simulink model "SquatTrotClimbRefinedDesign_Energy"  (R2025b)
settings: Solver=ode45  StartTime=0.0  StopTime=200  MaxStep=0.1  RelTol=0.01  AbsTol=0.01  EnableMultiTasking=on
undefined symbols (not defined in the file): waypoints, X, Y, Z
libraries: nesl_utility x26, Quadruped_Lib x22, sm_lib x19, slpidlib x2, robotalgslib x1, sharedtransform x1
(part 3 of 3)

== matlab function SquatTrotClimbRefinedDesign_Energy/Rear_left_gait/MATLAB Function2 ==
  data: t input; leg_id input; q_hip output; mode_cmd input
function q_hip = hip_motion_all_legs(t, leg_id, mode_cmd)
    T_squat_start = 101;
    T_walk_start  = 129;
    
    % --- [NEW] Absolute time node for ending the walk ---
    T_walk_end    = 169;  % Start braking and retracting legs exactly at 170 seconds
    
    if (mode_cmd == 1) || (t < T_squat_start)
        q_hip = 0; return;
    end
    
    % Phase 1: Squat and stand (102s - 130s)
    if t < T_walk_start
        tau = t - T_squat_start;
        q_stand = 0; q_squat = deg2rad(35);
        T1=3; T2=15; T3=3;
        
        if tau < T1
            u = tau/T1; 
            q_hip = (1-u)*q_stand + u*q_squat;
        elseif tau < T1+T2
            q_hip = q_squat;
        elseif tau < T1+T2+T3
            u = (tau-(T1+T2))/T3; 
            q_hip = (1-u)*q_squat + u*q_stand;
        else
            q_hip = 0; 
        end
        return;
    end
    
    % Phase 2: Walking logic (130s+)
    % Relative time starting from 130s
    t_phase2 = t - T_walk_start;
    
    % ================= Tunables (Hip) =================
    ang_hip_crouch = deg2rad(30);    
    hip_swing_amp  = deg2rad(9);     
    
    ang_fwd  = ang_hip_crouch - hip_swing_amp;  
    ang_back = ang_hip_crouch + hip_swing_amp;  
    
    % ================= Timing =================
    T_crouch = 2.0;              
    T_hold   = 3.0;              
    T_ramp   = 2.0;              
    T_cycle  = 1.8;
    duty     = 0.50;             
    
    % --- [NEW] Braking and recovery time periods ---
    T_ramp_down = 2.0;    % 170s - 172s: Take 2 seconds to slowly reduce stride amplitude to 0
    T_recover   = 3.0;    % 172s - 175s: After legs stop, take 3 seconds to smoothly stand up straight (return to 0 degrees)
    
    % ================= Phase offsets =================
    phase_offset = [0.0, 0.5, 0.0, 0.5];
    phi = phase_offset(leg_id + 1);
    
    % ================= Smooth interpolators =================
    smooth = @(x) (1 - cos(x * pi)) / 2;
    
    % ==========================================================
    % Stage 1 & 2: Crouch & Hold (relative to 130s) -> (130s ~ 135s)
    % ==========================================================
    if t_phase2 < T_crouch + T_hold
        s = smooth(min(t_phase2 / T_crouch, 1.0));
        q_hip = s * ang_hip_crouch;
        return;
    end
    
    % ==========================================================
    % Stage 3: Trot & Stop (All motions after 135s)
    % ==========================================================
    t_trot = t_phase2 - T_crouch - T_hold;
    phase = mod(t_trot / T_cycle + phi, 1.0);
    
    % --- 1. Calculate theoretical pure gait trajectory (keep your already tuned normal logic) ---
    if phase < duty
        % ===== STANCE =====
        s = smooth(phase / duty);
        hip_walk  = ang_fwd + s * (ang_back - ang_fwd); 
    else
        % ===== SWING =====
        s = (phase - duty) / (1.0 - duty);
        hip_walk  = ang_back + smooth(s) * (ang_fwd - ang_back);
    end
    
    % Extract the pure stepping swing amount
    swing_offset = hip_walk - ang_hip_crouch;
    
    % --- 2. Calculate stride amplitude envelope (controls how large the step is) ---
    if t < T_walk_end
        % 135s - 170s: Start and maintain full speed
        amp_walk = smooth(min(t_trot / T_ramp, 1.0));
    elseif t < T_walk_end + T_ramp_down
        % 170s - 172s: Stride amplitude gradually decreases until stopping in place
        tau_stop = t - T_walk_end;
        amp_walk = smooth(max(1.0 - (tau_stop / T_ramp_down), 0.0));
    else
        % After 172s: Legs completely stop stepping
        amp_walk = 0.0;
    end
    
    % --- 3. Calculate base crouch angle (controls body height) ---
    if t < T_walk_end + T_ramp_down
        % Before 172s: Maintain 30 degree crouch baseline
        base_hip = ang_hip_crouch;
    elseif t < T_walk_end + T_ramp_down + T_recover
        % 172s - 175s: Smoothly stand up from 30 degree crouch back to 0 degrees
        tau_rec = t - (T_walk_end + T_ramp_down);
        s_rec = smooth(min(tau_rec / T_recover, 1.0));
        base_hip = (1.0 - s_rec) * ang_hip_crouch;
    else
        % After 175s: Completely stand straight, lock at 0 degrees, and enter wheeled driving mode
        base_hip = 0.0;
    end
    
    % --- 4. Final output = Base posture + (Stride proportion * Swing amount) ---
    q_hip = base_hip + amp_walk * swing_offset;
end

== matlab function SquatTrotClimbRefinedDesign_Energy/Rear_left_gait/MATLAB Function4 ==
  data: t input; leg_id input; q_knee output; mode_cmd input
function q_knee = knee_motion_all_legs(t, leg_id, mode_cmd)
    % --- Time Node Definitions ---
    T_squat_start = 101;
    T_walk_start  = 129; 
    
    % --- [NEW] Absolute time node for ending the walk ---
    T_walk_end    = 169;  
    
    % Phase 0: Standby
    if (mode_cmd == 1) || (t < T_squat_start)
        q_knee = 0; return;
    end
    
    % Phase 1: Squat and stand (102-130s)
    if t < T_walk_start
        tau = t - T_squat_start;
        q_stand = 0; q_squat = -deg2rad(70);
        T1=3; T2=15; T3=3;
        
        if tau < T1
            u = tau/T1; 
            q_knee = (1-u)*q_stand + u*q_squat;
        elseif tau < T1+T2
            q_knee = q_squat;
        elseif tau < T1+T2+T3
            u = (tau-(T1+T2))/T3; 
            q_knee = (1-u)*q_squat + u*q_stand;
        else
            q_knee = 0; 
        end
        return;
    end
    
    % Phase 2: Walking logic (130s+)
    % Relative time starting from 130s
    t_phase2 = t - T_walk_start;
    
    % ================= Tunables (Knee) =================
    ang_crouch = deg2rad(-40);   % Base walking crouch angle
    ang_lift   = deg2rad(-8);    % Leg lift amplitude during swing
    ang_comp   = deg2rad(-3);    % Compression amplitude during stance
    
    % ================= Timing =================
    T_crouch = 2.0;              
    T_hold   = 3.0;              
    T_ramp   = 2.0;              
    T_cycle  = 1.8;
    duty     = 0.50;             
    
    % --- [NEW] Braking and recovery time periods ---
    T_ramp_down = 2.0;    % 170s - 172s: Take 2 seconds to slowly reduce the step amplitude to 0
    T_recover   = 3.0;    % 172s - 175s: After the legs stop, take 3 seconds to smoothly stand up straight (return to 0 degrees)
    
    % ================= Phase offsets =================
    phase_offset = [0.0, 0.5, 0.0, 0.5];
    phi = phase_offset(leg_id + 1);
    
    % ================= Smooth interpolators =================
    smooth = @(x) (1 - cos(x * pi)) / 2;
    bump   = @(x) (1 - cos(2 * x * pi)) / 2;
    
    % ==========================================================
    % Stage 1 & 2: Crouch & Hold (relative to 130s) -> (130s ~ 135s)
    % ==========================================================
    if t_phase2 < T_crouch + T_hold
        s = smooth(min(t_phase2 / T_crouch, 1.0));
        q_knee = s * ang_crouch;
        return;
    end
    
    % ==========================================================
    % Stage 3: Trot & Stop (All motions after 135s)
    % ==========================================================
    t_trot = t_phase2 - T_crouch - T_hold;
    phase = mod(t_trot / T_cycle + phi, 1.0);
    
    % --- 1. Calculate theoretical pure gait trajectory (keep calculating normally to prevent phase disruption from sudden cutoff) ---
    if phase < duty
        % ===== STANCE: foot on ground =====
        knee_walk = ang_crouch + sin((phase / duty) * pi) * ang_comp;
    else
        % ===== SWING: foot in air =====
        s = (phase - duty) / (1.0 - duty);
        knee_walk = ang_crouch + bump(s) * ang_lift;
    end
    
    % Extract the pure stepping flexion/extension amount
    swing_offset = knee_walk - ang_crouch;
    
    % --- 2. Calculate stride amplitude envelope (controls how large the step is) ---
    if t < T_walk_end
        % 135s - 170s: Start and maintain full-amplitude stepping
        amp_walk = smooth(min(t_trot / T_ramp, 1.0));
    elseif t < T_walk_end + T_ramp_down
        % 170s - 172s: Stride amplitude gradually decreases until stopping in place
        tau_stop = t - T_walk_end;
        amp_walk = smooth(max(1.0 - (tau_stop / T_ramp_down), 0.0));
    else
        % After 172s: Legs completely stop stepping
        amp_walk = 0.0;
    end
    
    % --- 3. Calculate base crouch angle (controls body height) ---
    if t < T_walk_end + T_ramp_down
        % Before 172s: Maintain -40 degree crouch baseline
        base_knee = ang_crouch;
    elseif t < T_walk_end + T_ramp_down + T_recover
        % 172s - 175s: Smoothly stand up from -40 degrees back to 0 degrees
        tau_rec = t - (T_walk_end + T_ramp_down);
        s_rec = smooth(min(tau_rec / T_recover, 1.0));
        base_knee = (1.0 - s_rec) * ang_crouch;
    else
        % After 175s: Completely stand straight, lock at 0 degrees, and enter wheeled driving mode
        base_knee = 0.0;
    end
    
    % --- 4. Final synthesis ---
    % Final output = Base knee angle + (Stride proportion * Additional flexion/extension amount)
    q_knee = base_knee + amp_walk * swing_offset;
end

== matlab function SquatTrotClimbRefinedDesign_Energy/Subsystem6/MATLAB Function1 ==
  data: v input; wL_cmd output; w input; T input; r input; wR_cmd output
function [wL_cmd, wR_cmd] = wheelSpeedCmd(v, w, T, r)
% v: linear velocity [m/s]
% w: yaw rate [rad/s]
% T: track width [m]
% r: wheel radius [m]

vL = v - 0.5*T*w;
vR = v + 0.5*T*w;

wL_cmd = vL / r;
wR_cmd = vR / r;
end

== matlab function SquatTrotClimbRefinedDesign_Energy/Subsystem6/MATLAB Function ==
  data: v input; delta output; w input; L input; v output
function [delta, v] = Diff2Ackermann(v, w, L)
% input: 
%   v - Linear velocity (m/s)
%   w - Angular velocity (rad/s)
%   L - Wheelbase (m)
%
% output:
%   delta - front wheel rotation angel (rad)
%   v     -  velocity(m/s)
if abs(v) < 1e-3
    delta = 0;
else
    delta = atan(L * w / v);   % pure pursuit function
end

== matlab function SquatTrotClimbRefinedDesign_Energy/Front_left_gait/MATLAB Function2 ==
  data: t input; leg_id input; q_hip output; mode_cmd input
function q_hip = hip_motion_all_legs(t, leg_id, mode_cmd)
    % --- Time Node Definitions ---
    T_squat_start = 101;
    T_walk_start  = 129;
    
    % --- Absolute time nodes for ending the walk and recovery ---
    T_walk_end    = 169;  % Start braking and retracting legs exactly at 170 seconds
    
    % --- [NEW] Stair climbing start time ---
    T_climb_start = 174;  
    
    if (mode_cmd == 1) || (t < T_squat_start)
        q_hip = 0; return;
    end
    
    % ==========================================================
    % Phase 1: Squat and stand (102s - 130s)
    % ==========================================================
    if t < T_walk_start
        tau = t - T_squat_start;
        q_stand = 0; q_squat = deg2rad(35);
        T1=3; T2=15; T3=3;
        
        if tau < T1
            u = tau/T1; 
            q_hip = (1-u)*q_stand + u*q_squat;
        elseif tau < T1+T2
            q_hip = q_squat;
        elseif tau < T1+T2+T3
            u = (tau-(T1+T2))/T3; 
            q_hip = (1-u)*q_squat + u*q_stand;
        else
            q_hip = 0; 
        end
        return;
    end
    
    % ==========================================================
    % Phase 2 & 3: Walking, Stopping & Recovering (130s - 175s)
    % ==========================================================
    if t < T_climb_start
        % Relative time starting from 130s
        t_phase2 = t - T_walk_start;
        
        % === Tunables (Hip) ===
        ang_hip_crouch = deg2rad(30);    
        hip_swing_amp  = deg2rad(9);     
        
        ang_fwd  = ang_hip_crouch - hip_swing_amp;  
        ang_back = ang_hip_crouch + hip_swing_amp;  
        
        % === Timing ===
        T_crouch = 2.0;              
        T_hold   = 3.0;              
        T_ramp   = 2.0;              
        T_cycle  = 1.8;
        duty     = 0.50;             
        
        % === Braking and recovery time periods ===
        T_ramp_down = 2.0;    % 170s - 172s: Take 2 seconds to slowly reduce stride amplitude to 0
        T_recover   = 3.0;    % 172s - 175s: After legs stop, take 3 seconds to smoothly stand up straight (return to 0 degrees)
        
        % === Phase offsets ===
        phase_offset = [0.0, 0.5, 0.0, 0.5];
        phi = phase_offset(leg_id + 1);
        
        % === Smooth interpolators ===
        smooth = @(x) (1 - cos(x * pi)) / 2;
        
        % --- Stage 1 & 2: Crouch & Hold (130s ~ 135s) ---
        if t_phase2 < T_crouch + T_hold
            s = smooth(min(t_phase2 / T_crouch, 1.0));
            q_hip = s * ang_hip_crouch;
            return;
        end
        
        % --- Stage 3: Trot & Stop (135s ~ 175s) ---
        t_trot = t_phase2 - T_crouch - T_hold;
        phase = mod(t_trot / T_cycle + phi, 1.0);
        
        % 1. Calculate theoretical pure gait trajectory
        if phase < duty
            s = smooth(phase / duty);
            hip_walk  = ang_fwd + s * (ang_back - ang_fwd); 
        else
            s = (phase - duty) / (1.0 - duty);
            hip_walk  = ang_back + smooth(s) * (ang_fwd - ang_back);
        end
        swing_offset = hip_walk - ang_hip_crouch;
        
        % 2. Calculate stride amplitude envelope
        if t < T_walk_end
            amp_walk = smooth(min(t_trot / T_ramp, 1.0));
        elseif t < T_walk_end + T_ramp_down
            tau_stop = t - T_walk_end;
            amp_walk = smooth(max(1.0 - (tau_stop / T_ramp_down), 0.0));
        else
            amp_walk = 0.0;
        end
        
        % 3. Calculate base crouch angle
        if t < T_walk_end + T_ramp_down
            base_hip = ang_hip_crouch;
        elseif t < T_walk_end + T_ramp_down + T_recover
            tau_rec = t - (T_walk_end + T_ramp_down);
            s_rec = smooth(min(tau_rec / T_recover, 1.0));
            base_hip = (1.0 - s_rec) * ang_hip_crouch;
        else
            base_hip = 0.0;
        end
        
        % 4. Final output
        q_hip = base_hip + amp_walk * swing_offset;
        return;
    end
    
    % ==========================================================
    % Phase 4: Stair Climbing Motion (175s+)
    % ==========================================================
    tau_climb = t - T_climb_start; 
    
    % Climbing Parameters
    q_stand = 0;             % Seamless transition starting from a straight standing posture (0 degrees)
    q_lift  = deg2rad(-30);  % [Lift] Negative value to lift up and clear the step
    q_step  = deg2rad(20);   % [Landing] Positive value to land on step, adapting to height diff
    
    % Time Allocation
    T_up   = 2.0;   % Duration to lift
    T_hold = 9.0;   % Hold in air (Allow time for rear wheels to drive forward)
    T_down = 2.0;   % Duration to lower
    
    if tau_climb < T_up
        % 1. Lift Leg (Swing Up)
        u = tau_climb / T_up;
        q_hip = (1-u)*q_stand + u*q_lift;
        
    elseif tau_climb < (T_up + T_hold)
        % 2. Maintain Height (Vehicle should move forward now)
        q_hip = q_lift;
        
    elseif tau_climb < (T_up + T_hold + T_down)
        % 3. Lower Leg (Land on the step)
        dt = tau_climb - (T_up + T_hold);
        u = dt / T_down;
        q_hip = (1-u)*q_lift + u*q_step;
        
    else
        % 4. Maintain Stance on Step
        % (Keep this pose until all legs are up, then reset to 0 together)
        q_hip = q_step;
    end
end

== matlab function SquatTrotClimbRefinedDesign_Energy/FR/MATLAB Function3 ==
  data: t input; torque output; w input
function torque = Front_Wheel_Optimized_Lock(t, w)
    % Optimized brake to avoid numerical stiffness
    T_lock   = 130;
    T_unlock = 175;  % [NEW] Unlock time node, restore driving state
    
    B_heavy = 1000;  % Lowered damping value; 1000 is usually enough to lock a 0.127m wheel
    w_threshold = 1; % Deadzone threshold (rad/s)
    
    % If before 130s (preparation/squat phase), or after 175s (resume driving phase)
    % Brake torque is 0, the wheel is in a free-rolling or motor-driven state
    if (t < T_lock) || (t >= T_unlock)
        torque = 0;
    else
        % 130s - 175s (Walking phase): Apply damping to lock the wheel
        if abs(w) > w_threshold
            torque = -B_heavy * w;
        else
            % At very low speeds, use smaller damping to reduce the burden on the solver
            torque = -B_heavy * 0.1 * w; 
        end
    end
end

== matlab function SquatTrotClimbRefinedDesign_Energy/Front_left_gait/MATLAB Function3 ==
  data: t input; leg_id input; q_knee output; mode_cmd input
function q_knee = knee_motion_all_legs(t, leg_id, mode_cmd)
    % --- Time Node Definitions ---
    T_squat_start = 101;
    T_walk_start  = 129; 
    
    % --- Absolute time nodes for ending the walk and recovery ---
    T_walk_end    = 169;  
    
    % --- [NEW] Stair climbing start time ---
    T_climb_start = 174;  
    
    % Phase 0: Standby
    if (mode_cmd == 1) || (t < T_squat_start)
        q_knee = 0; return;
    end
    
    % ==========================================================
    % Phase 1: Squat and stand (102-130s)
    % ==========================================================
    if t < T_walk_start
        tau = t - T_squat_start;
        q_stand = 0; q_squat = -deg2rad(70);
        T1=3; T2=15; T3=3;
        
        if tau < T1
            u = tau/T1; 
            q_knee = (1-u)*q_stand + u*q_squat;
        elseif tau < T1+T2
            q_knee = q_squat;
        elseif tau < T1+T2+T3
            u = (tau-(T1+T2))/T3; 
            q_knee = (1-u)*q_squat + u*q_stand;
        else
            q_knee = 0; 
        end
        return;
    end
    
    % ==========================================================
    % Phase 2 & 3: Walking, Stopping & Recovering (130s - 175s)
    % ==========================================================
    if t < T_climb_start
        % Relative time starting from 130s
        t_phase2 = t - T_walk_start;
        
        % === Tunables (Knee) ===
        ang_crouch = deg2rad(-40);   % Base walking crouch angle
        ang_lift   = deg2rad(-8);    % Leg lift amplitude during swing
        ang_comp   = deg2rad(-3);    % Compression amplitude during stance
        
        % === Timing ===
        T_crouch = 2.0;              
        T_hold   = 3.0;              
        T_ramp   = 2.0;              
        T_cycle  = 1.8;
        duty     = 0.50;             
        
        % === Braking and recovery time periods ===
        T_ramp_down = 2.0;    % 170s - 172s: Take 2 seconds to slowly reduce stride amplitude to 0
        T_recover   = 3.0;    % 172s - 175s: After legs stop, take 3 seconds to smoothly stand up straight (return to 0 degrees)
        
        % === Phase offsets ===
        phase_offset = [0.0, 0.5, 0.0, 0.5];
        phi = phase_offset(leg_id + 1);
        
        % === Smooth interpolators ===
        smooth = @(x) (1 - cos(x * pi)) / 2;
        bump   = @(x) (1 - cos(2 * x * pi)) / 2;
        
        % --- Stage 1 & 2: Crouch & Hold (130s ~ 135s) ---
        if t_phase2 < T_crouch + T_hold
            s = smooth(min(t_phase2 / T_crouch, 1.0));
            q_knee = s * ang_crouch;
            return;
        end
        
        % --- Stage 3: Trot & Stop (135s ~ 175s) ---
        t_trot = t_phase2 - T_crouch - T_hold;
        phase = mod(t_trot / T_cycle + phi, 1.0);
        
        % 1. Calculate theoretical pure gait trajectory
        if phase < duty
            knee_walk = ang_crouch + sin((phase / duty) * pi) * ang_comp;
        else
            s = (phase - duty) / (1.0 - duty);
            knee_walk = ang_crouch + bump(s) * ang_lift;
        end
        swing_offset = knee_walk - ang_crouch;
        
        % 2. Calculate stride amplitude envelope
        if t < T_walk_end
            amp_walk = smooth(min(t_trot / T_ramp, 1.0));
        elseif t < T_walk_end + T_ramp_down
            tau_stop = t - T_walk_end;
            amp_walk = smooth(max(1.0 - (tau_stop / T_ramp_down), 0.0));
        else
            amp_walk = 0.0;
        end
        
        % 3. Calculate base crouch angle
        if t < T_walk_end + T_ramp_down
            base_knee = ang_crouch;
        elseif t < T_walk_end + T_ramp_down + T_recover
            tau_rec = t - (T_walk_end + T_ramp_down);
            s_rec = smooth(min(tau_rec / T_recover, 1.0));
            base_knee = (1.0 - s_rec) * ang_crouch;
        else
            base_knee = 0.0;
        end
        
        % 4. Final synthesis
        q_knee = base_knee + amp_walk * swing_offset;
        return;
    end
    
    % ==========================================================
    % Phase 4: Stair Climbing Motion (175s+)
    % ==========================================================
    tau_climb = t - T_climb_start;
    
    % Climbing Parameters
    q_stand = 0;             % Seamless transition starting from a straight standing posture (0 degrees)
    q_lift  = deg2rad(-30);  % [Critical] Large knee bend to retract/lift the wheel
    q_step  = deg2rad(-90);  % [Landing] Land on step, slight bend for damping/buffering
    
    % Motion Timing Distribution
    T_up   = 2.0;
    T_hold = 9.0;
    T_down = 2.0;
    
    if tau_climb < T_up
        % 1. Lift Leg (Retraction)
        u = tau_climb / T_up;
        q_knee = (1-u)*q_stand + u*q_lift;
        
    elseif tau_climb < (T_up + T_hold)
        % 2. Hold High
        q_knee = q_lift;
        
    elseif tau_climb < (T_up + T_hold + T_down)
        % 3. Lower Leg (Placement)
        dt = tau_climb - (T_up + T_hold);
        u = dt / T_down;
        q_knee = (1-u)*q_lift + u*q_step;
        
    else
        % 4. Maintain stance on the step
        q_knee = q_step;
    end
end

== matlab function SquatTrotClimbRefinedDesign_Energy/FL/MATLAB Function3 ==
  data: t input; torque output; w input
function torque = Front_Wheel_Optimized_Lock(t, w)
    % Optimized brake to avoid numerical stiffness
    T_lock   = 130;
    T_unlock = 175;  % [NEW] Unlock time node, restore driving state
    
    B_heavy = 1000;  % Lowered damping value; 1000 is usually enough to lock a 0.127m wheel
    w_threshold = 1; % Deadzone threshold (rad/s)
    
    % If before 130s (preparation/squat phase), or after 175s (resume driving phase)
    % Brake torque is 0, the wheel is in a free-rolling or motor-driven state
    if (t < T_lock) || (t >= T_unlock)
        torque = 0;
    else
        % 130s - 175s (Walking phase): Apply damping to lock the wheel
        if abs(w) > w_threshold
            torque = -B_heavy * w;
        else
            % At very low speeds, use smaller damping to reduce the burden on the solver
            torque = -B_heavy * 0.1 * w; 
        end
    end
end

== matlab function SquatTrotClimbRefinedDesign_Energy/Front_right_gait/MATLAB Function1 ==
  data: t input; leg_id input; q_hip output; mode_cmd input
function q_hip = hip_FR_motion(t, leg_id, mode_cmd)
    % --- Time Node Definitions ---
    T_squat_start = 101;
    T_walk_start  = 129;
    
    % --- Absolute time node for ending the walk and recovery ---
    T_walk_end    = 169;  % Start braking and retracting legs exactly at 170 seconds
    
    % --- [EXCLUSIVE MODIFICATION] FR leg stair climbing start time (175s stand straight + 5s delay) ---
    T_climb_start = 179;  
    
    % Phase 0: Standby
    if (mode_cmd == 1) || (t < T_squat_start)
        q_hip = 0; return;
    end
    
    % ==========================================================
    % Phase 1: Squat and stand (102s - 130s)
    % ==========================================================
    if t < T_walk_start
        tau = t - T_squat_start;
        q_stand = 0; q_squat = deg2rad(35);
        T1=3; T2=15; T3=3;
        
        if tau < T1
            u = tau/T1; 
            q_hip = (1-u)*q_stand + u*q_squat;
        elseif tau < T1+T2
            q_hip = q_squat;
        elseif tau < T1+T2+T3
            u = (tau-(T1+T2))/T3; 
            q_hip = (1-u)*q_squat + u*q_stand;
        else
            q_hip = 0; 
        end
        return;
    end
    
    % ==========================================================
    % Phase 2 & 3: Walking, Stopping & Recovering (130s - 180s)
    % ==========================================================
    % Between 175s - 180s, the body stays upright (0 degrees) in "idle" mode,
    % waiting for the 180s mark to begin stair climbing.
    if t < T_climb_start
        t_phase2 = t - T_walk_start;
        
        % ================= Tunables (Hip) =================
        ang_hip_crouch = deg2rad(30);    
        hip_swing_amp  = deg2rad(9);     
        
        ang_fwd  = ang_hip_crouch - hip_swing_amp;  
        ang_back = ang_hip_crouch + hip_swing_amp;  
        
        % ================= Timing =================
        T_crouch = 2.0;              
        T_hold   = 3.0;              
        T_ramp   = 2.0;              
        T_cycle  = 1.8;
        duty     = 0.50;             
        
        % --- Braking and recovery time periods ---
        T_ramp_down = 2.0;    
        T_recover   = 3.0;    
        
        % ================= Phase offsets =================
        phase_offset = [0.0, 0.5, 0.0, 0.5];
        phi = phase_offset(leg_id + 1);
        
        smooth = @(x) (1 - cos(x * pi)) / 2;
        
        % --- Stage 1 & 2: Crouch & Hold (130s ~ 135s) ---
        if t_phase2 < T_crouch + T_hold
            s = smooth(min(t_phase2 / T_crouch, 1.0));
            q_hip = s * ang_hip_crouch;
            return;
        end
        
        % --- Stage 3: Trot & Stop ---
        t_trot = t_phase2 - T_crouch - T_hold;
        phase = mod(t_trot / T_cycle + phi, 1.0);
        
        % 1. Calculate theoretical pure gait trajectory
        if phase < duty
            s = smooth(phase / duty);
            hip_walk  = ang_fwd + s * (ang_back - ang_fwd); 
        else
            s = (phase - duty) / (1.0 - duty);
            hip_walk  = ang_back + smooth(s) * (ang_fwd - ang_back);
        end
        swing_offset = hip_walk - ang_hip_crouch;
        
        % 2. Calculate stride amplitude envelope
        if t < T_walk_end
            amp_walk = smooth(min(t_trot / T_ramp, 1.0));
        elseif t < T_walk_end + T_ramp_down
            tau_stop = t - T_walk_end;
            amp_walk = smooth(max(1.0 - (tau_stop / T_ramp_down), 0.0));
        else
            amp_walk = 0.0;
        end
        
        % 3. Calculate crouch baseline angle
        if t < T_walk_end + T_ramp_down
            base_hip = ang_hip_crouch;
        elseif t < T_walk_end + T_ramp_down + T_recover
            tau_rec = t - (T_walk_end + T_ramp_down);
            s_rec = smooth(min(tau_rec / T_recover, 1.0));
            base_hip = (1.0 - s_rec) * ang_hip_crouch;
        else
            base_hip = 0.0; % Outputs 0 during 175s - 180s for perfectly static standing
        end
        
        q_hip = base_hip + amp_walk * swing_offset;
        return;
    end
    
    % ==========================================================
    % Phase 4: Stair Climbing Motion (Starts at 180s for FR)
    % ==========================================================
    tau_climb = t - T_climb_start; 
    
    % Climbing Parameters
    q_stand = 0;
    q_lift  = deg2rad(-30);  % [Lift] Negative value to lift up and clear the step
    q_step  = deg2rad(20);   % [Landing] Positive value to land on step
    
    % --- [EXCLUSIVE MODIFICATION] Motion Timing Distribution ---
    T_up   = 2.0;   
    T_hold = 4.0;    % Shortened to 4s as per your setting
    T_down = 2.0;   
    
    if tau_climb < T_up
        % 1. Lift Leg (Swing Up)
        u = tau_climb / T_up;
        q_hip = (1-u)*q_stand + u*q_lift;
        
    elseif tau_climb < (T_up + T_hold)
        % 2. Maintain Height (Vehicle should move forward now)
        q_hip = q_lift;
        
    elseif tau_climb < (T_up + T_hold + T_down)
        % 3. Lower Leg (Land on the step)
        dt = tau_climb - (T_up + T_hold);
        u = dt / T_down;
        q_hip = (1-u)*q_lift + u*q_step;
        
    else
        % 4. Maintain Stance on Step
        q_hip = q_step;
    end
end

== matlab function SquatTrotClimbRefinedDesign_Energy/Front_right_gait/MATLAB Function4 ==
  data: t input; leg_id input; q_knee output; mode_cmd input
function q_knee = knee_FR_motion(t, leg_id, mode_cmd)
    % --- Time Node Definitions ---
    T_squat_start = 101;
    T_walk_start  = 129; 
    
    % --- Absolute time node for ending the walk and recovery ---
    T_walk_end    = 169;  
    
    % --- [EXCLUSIVE MODIFICATION] FR leg stair climbing start time (175s stand straight + 5s delay) ---
    T_climb_start = 179;  
    
    % Phase 0: Standby
    if (mode_cmd == 1) || (t < T_squat_start)
        q_knee = 0; return;
    end
    
    % ==========================================================
    % Phase 1: Squat and stand (102-130s)
    % ==========================================================
    if t < T_walk_start
        tau = t - T_squat_start;
        q_stand = 0; q_squat = -deg2rad(70);
        T1=3; T2=15; T3=3;
        
        if tau < T1
            u = tau/T1; 
            q_knee = (1-u)*q_stand + u*q_squat;
        elseif tau < T1+T2
            q_knee = q_squat;
        elseif tau < T1+T2+T3
            u = (tau-(T1+T2))/T3; 
            q_knee = (1-u)*q_squat + u*q_stand;
        else
            q_knee = 0; 
        end
        return;
    end
    
    % ==========================================================
    % Phase 2 & 3: Walking, Stopping & Recovering (130s - 180s)
    % ==========================================================
    % Note: Although it stands straight at 175s, in order to keep it waiting at 0 degrees 
    % between 175-180s, we extend the jurisdiction of this logic to T_climb_start (180s)
    if t < T_climb_start
        t_phase2 = t - T_walk_start;
        
        % ================= Tunables (Knee) =================
        ang_crouch = deg2rad(-40);   
        ang_lift   = deg2rad(-8);    
        ang_comp   = deg2rad(-3);    
        
        % ================= Timing =================
        T_crouch = 2.0;              
        T_hold   = 3.0;              
        T_ramp   = 2.0;              
        T_cycle  = 1.8;
        duty     = 0.50;             
        
        T_ramp_down = 2.0;    % 170s-172s brake
        T_recover   = 3.0;    % 172s-175s stand straight
        
        % ================= Phase offsets =================
        phase_offset = [0.0, 0.5, 0.0, 0.5];
        phi = phase_offset(leg_id + 1);
        
        smooth = @(x) (1 - cos(x * pi)) / 2;
        bump   = @(x) (1 - cos(2 * x * pi)) / 2;
        
        if t_phase2 < T_crouch + T_hold
            s = smooth(min(t_phase2 / T_crouch, 1.0));
            q_knee = s * ang_crouch;
            return;
        end
        
        t_trot = t_phase2 - T_crouch - T_hold;
        phase = mod(t_trot / T_cycle + phi, 1.0);
        
        if phase < duty
            knee_walk = ang_crouch + sin((phase / duty) * pi) * ang_comp;
        else
            s = (phase - duty) / (1.0 - duty);
            knee_walk = ang_crouch + bump(s) * ang_lift;
        end
        swing_offset = knee_walk - ang_crouch;
        
        if t < T_walk_end
            amp_walk = smooth(min(t_trot / T_ramp, 1.0));
        elseif t < T_walk_end + T_ramp_down
            tau_stop = t - T_walk_end;
            amp_walk = smooth(max(1.0 - (tau_stop / T_ramp_down), 0.0));
        else
            amp_walk = 0.0;
        end
        
        if t < T_walk_end + T_ramp_down
            base_knee = ang_crouch;
        elseif t < T_walk_end + T_ramp_down + T_recover
            tau_rec = t - (T_walk_end + T_ramp_down);
            s_rec = smooth(min(tau_rec / T_recover, 1.0));
            base_knee = (1.0 - s_rec) * ang_crouch;
        else
            base_knee = 0.0; % Between 175s and 180s, this will continuously output 0, perfectly implementing the wait!
        end
        
        q_knee = base_knee + amp_walk * swing_offset;
        return;
    end
    
    % ==========================================================
    % Phase 4: Stair Climbing Motion (Starts at 180s for FR)
    % ==========================================================
    tau_climb = t - T_climb_start;
    
    % Climbing Parameters
    q_stand = 0;
    q_lift  = deg2rad(-45);  
    q_step  = deg2rad(-90);  
    
    % --- [EXCLUSIVE MODIFICATION] Motion Timing Distribution ---
    T_up   = 2.0;
    T_hold = 4.0;    % Shortened to 4s according to your setting
    T_down = 2.0;
    
    if tau_climb < T_up
        % 1. Lift Leg (Retraction)
        u = tau_climb / T_up;
        q_knee = (1-u)*q_stand + u*q_lift;
        
    elseif tau_climb < (T_up + T_hold)
        % 2. Hold High
        q_knee = q_lift;
        
    elseif tau_climb < (T_up + T_hold + T_down)
        % 3. Lower Leg (Placement)
        dt = tau_climb - (T_up + T_hold);
        u = dt / T_down;
        q_knee = (1-u)*q_lift + u*q_step;
        
    else
        % 4. Maintain stance on the step
        q_knee = q_step;
    end
end

== matlab function SquatTrotClimbRefinedDesign_Energy/Rear_right_gait/MATLAB Function2 ==
  data: t input; leg_id input; q_hip output; mode_cmd input
function q_hip = hip_motion_all_legs(t, leg_id, mode_cmd)
    T_squat_start = 101;
    T_walk_start  = 129;
    
    % --- [NEW] Absolute time node for ending the walk ---
    T_walk_end    = 169;  % Start braking and retracting legs exactly at 170 seconds
    
    if (mode_cmd == 1) || (t < T_squat_start)
        q_hip = 0; return;
    end
    
    % Phase 1: Squat and stand (102s - 130s)
    if t < T_walk_start
        tau = t - T_squat_start;
        q_stand = 0; q_squat = deg2rad(35);
        T1=3; T2=15; T3=3;
        
        if tau < T1
            u = tau/T1; 
            q_hip = (1-u)*q_stand + u*q_squat;
        elseif tau < T1+T2
            q_hip = q_squat;
        elseif tau < T1+T2+T3
            u = (tau-(T1+T2))/T3; 
            q_hip = (1-u)*q_squat + u*q_stand;
        else
            q_hip = 0; 
        end
        return;
    end
    
    % Phase 2: Walking logic (130s+)
    % Relative time starting from 130s
    t_phase2 = t - T_walk_start;
    
    % ================= Tunables (Hip) =================
    ang_hip_crouch = deg2rad(30);    
    hip_swing_amp  = deg2rad(9);     
    
    ang_fwd  = ang_hip_crouch - hip_swing_amp;  
    ang_back = ang_hip_crouch + hip_swing_amp;  
    
    % ================= Timing =================
    T_crouch = 2.0;              
    T_hold   = 3.0;              
    T_ramp   = 2.0;              
    T_cycle  = 1.8;
    duty     = 0.50;             
    
    % --- [NEW] Braking and recovery time periods ---
    T_ramp_down = 2.0;    % 170s - 172s: Take 2 seconds to slowly reduce stride amplitude to 0
    T_recover   = 3.0;    % 172s - 175s: After legs stop, take 3 seconds to smoothly stand up straight (return to 0 degrees)
    
    % ================= Phase offsets =================
    phase_offset = [0.0, 0.5, 0.0, 0.5];
    phi = phase_offset(leg_id + 1);
    
    % ================= Smooth interpolators =================
    smooth = @(x) (1 - cos(x * pi)) / 2;
    
    % ==========================================================
    % Stage 1 & 2: Crouch & Hold (relative to 130s) -> (130s ~ 135s)
    % ==========================================================
    if t_phase2 < T_crouch + T_hold
        s = smooth(min(t_phase2 / T_crouch, 1.0));
        q_hip = s * ang_hip_crouch;
        return;
    end
    
    % ==========================================================
    % Stage 3: Trot & Stop (All motions after 135s)
    % ==========================================================
    t_trot = t_phase2 - T_crouch - T_hold;
    phase = mod(t_trot / T_cycle + phi, 1.0);
    
    % --- 1. Calculate theoretical pure gait trajectory (keep your already tuned normal logic) ---
    if phase < duty
        % ===== STANCE =====
        s = smooth(phase / duty);
        hip_walk  = ang_fwd + s * (ang_back - ang_fwd); 
    else
        % ===== SWING =====
        s = (phase - duty) / (1.0 - duty);
        hip_walk  = ang_back + smooth(s) * (ang_fwd - ang_back);
    end
    
    % Extract the pure stepping swing amount
    swing_offset = hip_walk - ang_hip_crouch;
    
    % --- 2. Calculate stride amplitude envelope (controls how large the step is) ---
    if t < T_walk_end
        % 135s - 170s: Start and maintain full speed
        amp_walk = smooth(min(t_trot / T_ramp, 1.0));
    elseif t < T_walk_end + T_ramp_down
        % 170s - 172s: Stride amplitude gradually decreases until stopping in place
        tau_stop = t - T_walk_end;
        amp_walk = smooth(max(1.0 - (tau_stop / T_ramp_down), 0.0));
    else
        % After 172s: Legs completely stop stepping
        amp_walk = 0.0;
    end
    
    % --- 3. Calculate base crouch angle (controls body height) ---
    if t < T_walk_end + T_ramp_down
        % Before 172s: Maintain 30 degree crouch baseline
        base_hip = ang_hip_crouch;
    elseif t < T_walk_end + T_ramp_down + T_recover
        % 172s - 175s: Smoothly stand up from 30 degree crouch back to 0 degrees
        tau_rec = t - (T_walk_end + T_ramp_down);
        s_rec = smooth(min(tau_rec / T_recover, 1.0));
        base_hip = (1.0 - s_rec) * ang_hip_crouch;
    else
        % After 175s: Completely stand straight, lock at 0 degrees, and enter wheeled driving mode
        base_hip = 0.0;
    end
    
    % --- 4. Final output = Base posture + (Stride proportion * Swing amount) ---
    q_hip = base_hip + amp_walk * swing_offset;
end

== matlab function SquatTrotClimbRefinedDesign_Energy/Rear_right_gait/MATLAB Function3 ==
  data: t input; leg_id input; q_knee output; mode_cmd input
function q_knee = knee_motion_all_legs(t, leg_id, mode_cmd)
    % --- Time Node Definitions ---
    T_squat_start = 101;
    T_walk_start  = 129; 
    
    % --- [NEW] Absolute time node for ending the walk ---
    T_walk_end    = 169;  
    
    % Phase 0: Standby
    if (mode_cmd == 1) || (t < T_squat_start)
        q_knee = 0; return;
    end
    
    % Phase 1: Squat and stand (102-130s)
    if t < T_walk_start
        tau = t - T_squat_start;
        q_stand = 0; q_squat = -deg2rad(70);
        T1=3; T2=15; T3=3;
        
        if tau < T1
            u = tau/T1; 
            q_knee = (1-u)*q_stand + u*q_squat;
        elseif tau < T1+T2
            q_knee = q_squat;
        elseif tau < T1+T2+T3
            u = (tau-(T1+T2))/T3; 
            q_knee = (1-u)*q_squat + u*q_stand;
        else
            q_knee = 0; 
        end
        return;
    end
    
    % Phase 2: Walking logic (130s+)
    % Relative time starting from 130s
    t_phase2 = t - T_walk_start;
    
    % ================= Tunables (Knee) =================
    ang_crouch = deg2rad(-40);   % Base walking crouch angle
    ang_lift   = deg2rad(-8);    % Leg lift amplitude during swing
    ang_comp   = deg2rad(-3);    % Compression amplitude during stance
    
    % ================= Timing =================
    T_crouch = 2.0;              
    T_hold   = 3.0;              
    T_ramp   = 2.0;              
    T_cycle  = 1.8;
    duty     = 0.50;             
    
    % --- [NEW] Braking and recovery time periods ---
    T_ramp_down = 2.0;    % 170s - 172s: Take 2 seconds to slowly reduce the step amplitude to 0
    T_recover   = 3.0;    % 172s - 175s: After the legs stop, take 3 seconds to smoothly stand up straight (return to 0 degrees)
    
    % ================= Phase offsets =================
    phase_offset = [0.0, 0.5, 0.0, 0.5];
    phi = phase_offset(leg_id + 1);
    
    % ================= Smooth interpolators =================
    smooth = @(x) (1 - cos(x * pi)) / 2;
    bump   = @(x) (1 - cos(2 * x * pi)) / 2;
    
    % ==========================================================
    % Stage 1 & 2: Crouch & Hold (relative to 130s) -> (130s ~ 135s)
    % ==========================================================
    if t_phase2 < T_crouch + T_hold
        s = smooth(min(t_phase2 / T_crouch, 1.0));
        q_knee = s * ang_crouch;
        return;
    end
    
    % ==========================================================
    % Stage 3: Trot & Stop (All motions after 135s)
    % ==========================================================
    t_trot = t_phase2 - T_crouch - T_hold;
    phase = mod(t_trot / T_cycle + phi, 1.0);
    
    % --- 1. Calculate theoretical pure gait trajectory (keep calculating normally to prevent phase disruption from sudden cutoff) ---
    if phase < duty
        % ===== STANCE: foot on ground =====
        knee_walk = ang_crouch + sin((phase / duty) * pi) * ang_comp;
    else
        % ===== SWING: foot in air =====
        s = (phase - duty) / (1.0 - duty);
        knee_walk = ang_crouch + bump(s) * ang_lift;
    end
    
    % Extract the pure stepping flexion/extension amount
    swing_offset = knee_walk - ang_crouch;
    
    % --- 2. Calculate stride amplitude envelope (controls how large the step is) ---
    if t < T_walk_end
        % 135s - 170s: Start and maintain full-amplitude stepping
        amp_walk = smooth(min(t_trot / T_ramp, 1.0));
    elseif t < T_walk_end + T_ramp_down
        % 170s - 172s: Stride amplitude gradually decreases until stopping in place
        tau_stop = t - T_walk_end;
        amp_walk = smooth(max(1.0 - (tau_stop / T_ramp_down), 0.0));
    else
        % After 172s: Legs completely stop stepping
        amp_walk = 0.0;
    end
    
    % --- 3. Calculate base crouch angle (controls body height) ---
    if t < T_walk_end + T_ramp_down
        % Before 172s: Maintain -40 degree crouch baseline
        base_knee = ang_crouch;
    elseif t < T_walk_end + T_ramp_down + T_recover
        % 172s - 175s: Smoothly stand up from -40 degrees back to 0 degrees
        tau_rec = t - (T_walk_end + T_ramp_down);
        s_rec = smooth(min(tau_rec / T_recover, 1.0));
        base_knee = (1.0 - s_rec) * ang_crouch;
    else
        % After 175s: Completely stand straight, lock at 0 degrees, and enter wheeled driving mode
        base_knee = 0.0;
    end
    
    % --- 4. Final synthesis ---
    % Final output = Base knee angle + (Stride proportion * Additional flexion/extension amount)
    q_knee = base_knee + amp_walk * swing_offset;
end
